simulink model "clawbot_planner"  (R2020b)
settings: Solver=VariableStepAuto  StartTime=0.0  StopTime=100  MaxStep=0.1  RelTol=1e-3
model workspace (MAT data in the model file):
  objPose = [-3 -4 0]
  pickup = 1
undefined symbols (not defined in the file): boxPose, goalPose, n_box, startPose, waypoints, X, Y, Z
libraries: sm_lib x10, robotics_pg_exp_pack x6, nesl_utility x5
settings Model: PacingRate=2  OrderedModelArguments=off  Creator=fciriell  LastModifiedBy=philip
settings ExplorerConfigSet: InternalSimMechanicsExplorerSettings="<ExplorerConfiguration><canonicalview>default</canonicalview><AnimationSetting><BasePlaybackSpeed>1.0</BasePlaybackSpeed><PlaybackSpeedFactor>1.0</PlaybackSpeedFactor></AnimationSetting><TilePanel><TileInfo><Tiles Columns=\"2\" Count=\"2\" Rows=\"1\"><Column Weight=\"0.4995\"/><Column Weight=\"0.5005\"/><Row Weight=\"1\"/><Tile Height=\"1\" Width=\"1\" X=\"0\" Y=\"0\"/><Tile Height=\"1\" Width=\"1\" X=\"1\" Y=\"0\"/></Tiles></TileInfo><SceneInfo><SceneViewer><BGColor><R>0.800000011920928955</R><G>1</G><B>1</B></BGColor><Camera><DoPerspective>off</DoPerspective><Position><X>-2157.55283921657792</X><Y>-624.799824111750013</Y><Z>101.181168331954723</Z></Position><Center><X>0.446420361421132839</X><Y>8.2063001014053043</Y><Z>-0.139153976130387491</Z></Center><Up><X>-0.0243727538639528785</X><Y>0.238484651328139785</Y><Z>0.970840378203329246</Z></Up><ViewLimDist>1</ViewLimDist><YLim>1.44671838529622754</YLim><XLim>1.08018402928996848</XLim></Camera></SceneViewer><SceneViewer><BGColor><R>0.800000011920928955</R><G>1</G><B>1</B></BGColor><Camera><DoPerspective>on</DoPerspective><Position><X>4.31003215901698322</X><Y>10.0399967053635688</Y><Z>0.101600000000000093</Z></Position><Center><X>3.31158832209072962</X><Y>9.99016648666538565</Y><Z>0.126637048717288314</Z></Center><Up><X>0.02500592574512428</X><Y>0.0012479928289858</Y><Z>0.999686523962150853</Z></Up><ViewLimDist>1</ViewLimDist><YLim>0.466307658154998583</YLim><XLim>0.348165952817071078</XLim></Camera></SceneViewer></SceneInfo></TilePanel><MechEditorPanel><Cameras><Camera><Id>Camera1</Id><Value><Name>pov</Name><NativeCamera><PositionTrackingFeature>ClawBot_Kinematic_Model_with_spherical_contact_gripper.Chassis.Vehicle_Base.Frame2</PositionTrackingFeature><CenterTrackingFeature>ClawBot_Kinematic_Model_with_spherical_contact_gripper.Claw_Arm.Claw_Base.Claw_Mount.Frame1</CenterTrackingFeature><UpVectorTrackingFeature>ClawBot_Kinematic_Model_with_spherical_contact_gripper.Claw_Arm.Claw_Base.Claw_Mount.Frame1</UpVectorTrackingFeature><CenterTrackingOrigin>off</CenterTrackingOrigin><CenterTrackingDirection>+Y</CenterTrackingDirection><UpVectorTrackingDirection>+X</UpVectorTrackingDirection></NativeCamera></Value></Camera><Camera><Id>Camera2</Id><Value><Name>topview</Name><NativeCamera><PositionKeyframeSet><Keyframe><Time>150</Time><Value><X>6.1546883145524589e-08</X><Y>-4.7109925072064129e-08</Y><Z>4.4114050188881766</Z></Value></Keyframe></PositionKeyframeSet><CenterKeyframeSet><Keyframe><Time>150</Time><Value><X>6.1546883145524589e-08</X><Y>-4.7109925072064129e-08</Y><Z>0.00050000002374872565</Z></Value></Keyframe></CenterKeyframeSet><UpVectorKeyframeSet><Keyframe><Time>150</Time><Value><X>0</X><Y>1</Y><Z>-0</Z></Value></Keyframe></UpVectorKeyframeSet></NativeCamera></Value></Camera></Cameras><GfxPanelCameraMap><MapElement CameraMLId=\"Camera1\" GfxPanelIndex=\"1\"/></GfxPanelCameraMap><VideoCreator><PlaybackSpeedRatio>1.0</PlaybackSpeedRatio><FrameRate>30</FrameRate><VideoFormat>Motion JPEG AVI</VideoFormat><FrameSize>auto</FrameSize></VideoCreator></MechEditorPanel></ExplorerConfiguration>"

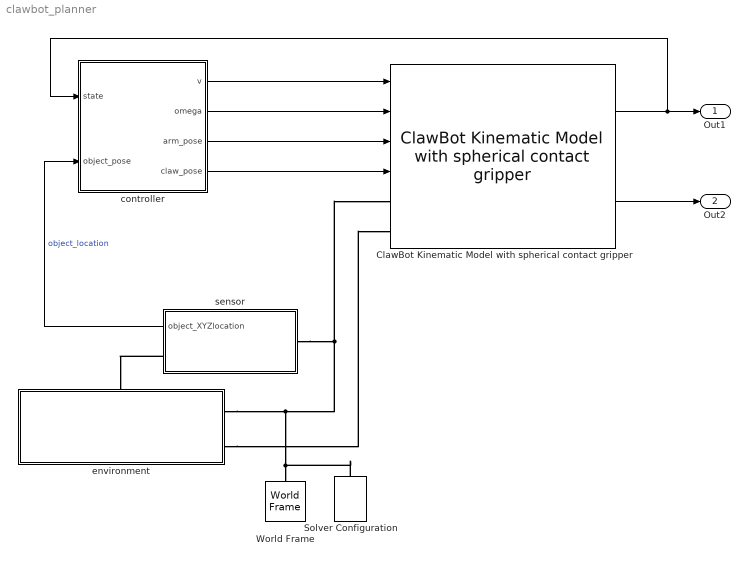
== system clawbot_planner ==
  ClawBot Kinematic Model with spherical contact gripper : robotics_pg_exp_pack/Robot Models/Clawbot/ClawBot Kinematic Model with spherical contact gripper  pose=startPose  k_contact=2*2.5*981  b_contact=sqrt(2*2.5*981)  x_contact=1e-2  u_statfric=10  u_dynfric=10  crit_vel_fric=1e-3  radius_contact_point=10  sensorTs=-1
      settings: SourceProductName=Robotics Playground Expansion Pack
  Solver Configuration : nesl_utility/Solver Configuration  PhysicalDomain=network_engine_domain  SubClassName=solver  LeftPortType=input  RightPortType=generic  Tones=[]  Harmonics=[]  SimulateNoise=off  Profile=off  UseLocalSampling=off  EnableSwitchedLinearOptims=on  FrequencyDomain=off  UseCCode=off  RelTol=0.001  AbsTol=1e-06  MinStep=1e-09  ToWorkspace=off  RevertToSquareIcSolve=off  NumHomotopyIterations=100  PhasorMode=off  PhasorModeNumHarmonics=1  DoDC=off  ResidualTolerance=1e-09  UseLocalSolver=off  LocalSolverChoice=NE_BACKWARD_EULER_ADVANCER  LocalSolverSampleTime=0.001  DoFixedCost=off  MaxNonlinIter=3  MaxModeIter=2  ComputeImpulses=off  ImpulseIterations=2  LinearAlgebra=auto  EquationFormulation=NE_TIME_EF  DelaysMemoryBudget=1024  AutomaticFiltering=on  FilteringTimeConstant=0.001  PartitionStorageMethod=AS_NEEDED  PartitionMemoryBudget=1024  PartitionMethod=ROBUST
  World Frame : sm_lib/Frames and Transforms/World Frame
  controller : Subsystem
  environment : Subsystem
      settings: PortSchema="{\"entries\":[{\"content\":{\"sides\":[{\"content\":{\"connectorIds\":[]},\"type\":\"ConnectorPlacement.EquallySpacedRectSide\",\"uuid\":\"883eba9b-41a6-4158-bc00-14a83777f32f\"},{\"content\":{\"connectorIds\":[\"RConn1\",\"RConn2\"],\"side\":\"RIGHT\"},\"type\":\"ConnectorPlacement.EquallySpacedRectSide\",\"uuid\":\"b95afd35-d391-4cad-9c3e-31548b5bac4e\"},{\"content\":{\"connectorIds\":[\"LConn1\"],\"side\":\"TOP\"},\"type\":\"ConnectorPlacement.EquallySpacedRectSide\",\"uuid\":\"0d35fa8f-0aa6-49ea-bb20-39be00b87579\"}]},\"type\":\"ConnectorPlacement.EquallySpacedConnector\",\"uuid\":\"10348ddd-2367-47d6-bad2-8db5a122cc9e\"}],\"packageUris\":[\"http://schema.mathworks.com/mf0/Connector/19700101\"],\"version\":\"1.0\"}"
  sensor : Subsystem
  Out1 : Outport
  Out2 : Outport  Port=2
  wires:
  sensor/1(object_XYZlocation) -> controller/2(object_pose)  "object_location"
  ClawBot Kinematic Model with spherical contact gripper/2 -> Out2/1
  ClawBot Kinematic Model with spherical contact gripper/1 -> controller/1(state), Out1/1
  controller/1(v) -> ClawBot Kinematic Model with spherical contact gripper/1
  controller/3(arm_pose) -> ClawBot Kinematic Model with spherical contact gripper/3
  controller/4(claw_pose) -> ClawBot Kinematic Model with spherical contact gripper/4
  controller/2(omega) -> ClawBot Kinematic Model with spherical contact gripper/2
  connections:
  environment/RConn1 -- Solver Configuration/RConn1 -- World Frame/RConn1 -- ClawBot Kinematic Model with spherical contact gripper/LConn1 -- sensor/LConn1
  environment/RConn2 -- ClawBot Kinematic Model with spherical contact gripper/LConn2
  sensor/RConn1 -- environment/LConn1

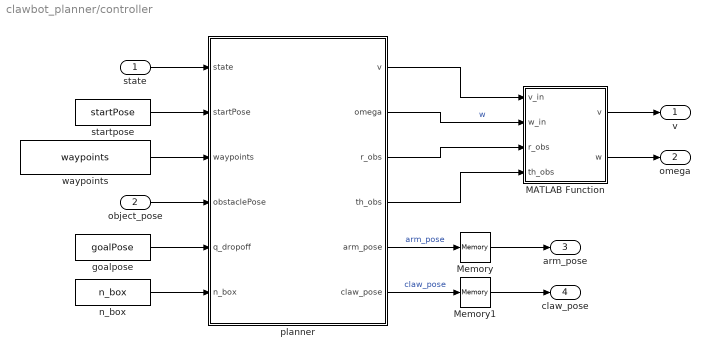
== system clawbot_planner/controller ==
  state : Inport
  object_pose : Inport  Port=2
  MATLAB Function : MATLAB Function  TreatAsAtomicUnit=on
  "Memory " : Memory
  Memory1 : Memory
  goalpose : Constant  Value=goalPose  SampleTime=0.01
  n_box : Constant  Value=n_box  SampleTime=0.01
  planner : Stateflow chart  TreatAsAtomicUnit=on
      settings: PortSchema="{\"entries\":[{\"content\":{\"sides\":[{\"content\":{\"connectorIds\":[\"In1\",\"In2\",\"In3\",\"In4\",\"In5\",\"In6\"]},\"type\":\"ConnectorPlacement.EquallySpacedRectSide\",\"uuid\":\"4907e7b4-59f6-4e30-9dc7-cd38531777e1\"},{\"content\":{\"connectorIds\":[\"Out1\",\"Out2\",\"Out6\",\"Out5\",\"Out3\",\"Out4\"],\"side\":\"RIGHT\"},\"type\":\"ConnectorPlacement.EquallySpacedRectSide\",\"uuid\":\"27f4ca00-c645-4624-ac98-a2a144dd84bb\"},{\"content\":{\"connectorIds\":[],\"side\":\"TOP\"},\"type\":\"ConnectorPlacement.EquallySpacedRectSide\",\"uuid\":\"2e3861bb-acf9-4584-a82a-efca55bff57a\"},{\"content\":{\"connectorIds\":[],\"side\":\"HIDDEN\"},\"type\":\"ConnectorPlacement.EquallySpacedRectSide\",\"uuid\":\"c95c31ea-85f8-4402-96cd-52bc89f7c1df\"}]},\"type\":\"ConnectorPlacement.EquallySpacedConnector\",\"uuid\":\"fce2e92a-f6ab-431e-a92c-b0146e5459eb\"}],\"packageUris\":[\"http://schema.mathworks.com/mf0/Connector/R2020b\"],\"version\":\"1.0\"}"
  startpose : Constant  Value=startPose  SampleTime=0.01
  waypoints : Constant  Value=waypoints  SampleTime=0.01
  v : Outport
  omega : Outport  Port=2
  arm_pose : Outport  Port=3
  claw_pose : Outport  Port=4
  wires:
  planner/4(claw_pose) -> Memory1/1  "claw_pose"
  planner/3(arm_pose) -> "Memory "/1  "arm_pose"
  Memory1/1 -> claw_pose/1
  "Memory "/1 -> arm_pose/1
  planner/1(v) -> MATLAB Function/1(v_in)
  goalpose/1 -> planner/5(q_dropoff)
  state/1 -> planner/1(state)
  startpose/1 -> planner/2(startPose)
  waypoints/1 -> planner/3(waypoints)
  object_pose/1 -> planner/4(obstaclePose)
  n_box/1 -> planner/6(n_box)
  MATLAB Function/2(w) -> omega/1
  planner/5(th_obs) -> MATLAB Function/4(th_obs)
  planner/6(r_obs) -> MATLAB Function/3(r_obs)
  planner/2(omega) -> MATLAB Function/2(w_in)  "w"
  MATLAB Function/1(v) -> v/1

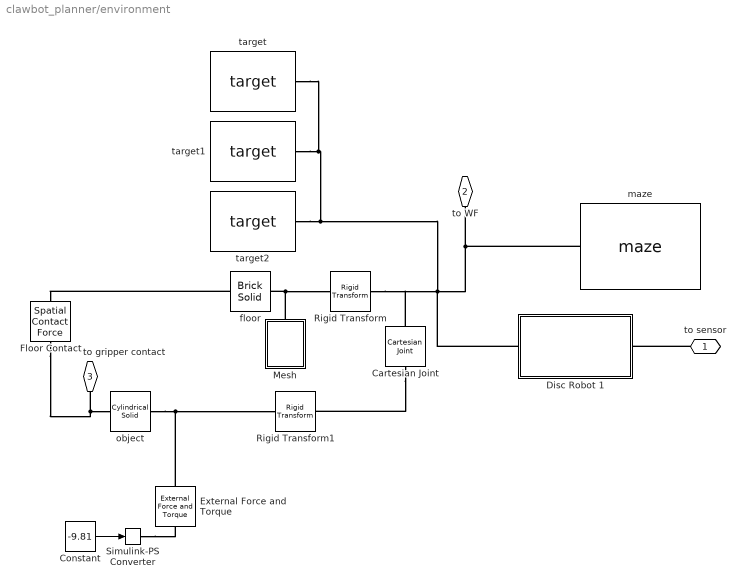
== system clawbot_planner/environment ==
  Cartesian Joint : sm_lib/Joints/Cartesian Joint  JointMode=Normal  SenseConstraintForce=off  SenseConstraintForceX=off  SenseConstraintForceY=off  SenseConstraintForceZ=off  SenseConstraintTorque=off  SenseConstraintTorqueX=off  SenseConstraintTorqueY=off  SenseConstraintTorqueZ=off  SenseTotalForce=off  SenseTotalForceX=off  SenseTotalForceY=off  SenseTotalForceZ=off  SenseTotalTorque=off  SenseTotalTorqueX=off  SenseTotalTorqueY=off  SenseTotalTorqueZ=off  CompositeWrenchDir=FollowerOnBase  CompositeWrenchFrame=BaseFrame  PxEquilibriumPosition=0  PxEquilibriumPositionUnits=m  PxSpringStiffness=1e-1  PxSpringStiffnessUnits=N/m  PxDampingCoefficient=1e-2  PxDampingCoefficientUnits=N/(m/s)  PxTorqueActuationMode=NoTorque  PxMotionActuationMode=ComputedMotion  PxSensePosition=off  PxSenseVelocity=off  PxSenseAcceleration=off  PxSenseTorqueForce=off  PxSenseLowerLimitTorqueForce=off  PxSenseUpperLimitTorqueForce=off  PxLowerLimitSpecify=off  PxLowerLimitBound=-1  PxLowerLimitBoundUnits=m  PxLowerLimitStiffness=1e6  PxLowerLimitStiffnessUnits=N/m  PxLowerLimitDamping=1e3  PxLowerLimitDampingUnits=N/(m/s)  PxLowerLimitTransitionRegionWidth=1e-4  PxLowerLimitTransitionRegionWidthUnits=m  PxUpperLimitSpecify=off  PxUpperLimitBound=1  PxUpperLimitBoundUnits=m  PxUpperLimitStiffness=1e6  PxUpperLimitStiffnessUnits=N/m  PxUpperLimitDamping=1e3  PxUpperLimitDampingUnits=N/(m/s)  PxUpperLimitTransitionRegionWidth=1e-4  PxUpperLimitTransitionRegionWidthUnits=m  PxPositionTargetSpecify=off  PxPositionTargetPriority=High  PxPositionTargetValue=0  PxPositionTargetValueUnits=m  PxVelocityTargetSpecify=off  PxVelocityTargetPriority=High  PxVelocityTargetValue=0  PxVelocityTargetValueUnits=m/s  PyEquilibriumPosition=0  PyEquilibriumPositionUnits=m  PySpringStiffness=1e-1  PySpringStiffnessUnits=N/m  PyDampingCoefficient=1e-2  PyDampingCoefficientUnits=N/(m/s)  PyTorqueActuationMode=NoTorque  PyMotionActuationMode=ComputedMotion  PySensePosition=off  PySenseVelocity=off  PySenseAcceleration=off  PySenseTorqueForce=off  PySenseLowerLimitTorqueForce=off  PySenseUpperLimitTorqueForce=off  PyLowerLimitSpecify=off  PyLowerLimitBound=-1  PyLowerLimitBoundUnits=m  PyLowerLimitStiffness=1e6  PyLowerLimitStiffnessUnits=N/m  PyLowerLimitDamping=1e3  PyLowerLimitDampingUnits=N/(m/s)  PyLowerLimitTransitionRegionWidth=1e-4  PyLowerLimitTransitionRegionWidthUnits=m  PyUpperLimitSpecify=off  PyUpperLimitBound=1  PyUpperLimitBoundUnits=m  PyUpperLimitStiffness=1e6  PyUpperLimitStiffnessUnits=N/m  PyUpperLimitDamping=1e3  PyUpperLimitDampingUnits=N/(m/s)  PyUpperLimitTransitionRegionWidth=1e-4  PyUpperLimitTransitionRegionWidthUnits=m  PyPositionTargetSpecify=off  PyPositionTargetPriority=High  PyPositionTargetValue=0  PyPositionTargetValueUnits=m  PyVelocityTargetSpecify=off  PyVelocityTargetPriority=High  PyVelocityTargetValue=0  PyVelocityTargetValueUnits=m/s  PzEquilibriumPosition=0  PzEquilibriumPositionUnits=m  PzSpringStiffness=1e-1  PzSpringStiffnessUnits=N/m  PzDampingCoefficient=1e-2  PzDampingCoefficientUnits=N/(m/s)  PzTorqueActuationMode=NoTorque  PzMotionActuationMode=ComputedMotion  PzSensePosition=off  PzSenseVelocity=off  PzSenseAcceleration=off  PzSenseTorqueForce=off  PzSenseLowerLimitTorqueForce=off  PzSenseUpperLimitTorqueForce=off  PzLowerLimitSpecify=off  PzLowerLimitBound=-1  PzLowerLimitBoundUnits=m  PzLowerLimitStiffness=1e6  PzLowerLimitStiffnessUnits=N/m  PzLowerLimitDamping=1e3  PzLowerLimitDampingUnits=N/(m/s)  PzLowerLimitTransitionRegionWidth=1e-4  PzLowerLimitTransitionRegionWidthUnits=m  PzUpperLimitSpecify=off  PzUpperLimitBound=1  PzUpperLimitBoundUnits=m  PzUpperLimitStiffness=1e6  PzUpperLimitStiffnessUnits=N/m  PzUpperLimitDamping=1e3  PzUpperLimitDampingUnits=N/(m/s)  PzUpperLimitTransitionRegionWidth=1e-4  PzUpperLimitTransitionRegionWidthUnits=m  PzPositionTargetSpecify=off  PzPositionTargetPriority=High  PzPositionTargetValue=0  PzPositionTargetValueUnits=m  PzVelocityTargetSpecify=off  PzVelocityTargetPriority=High  PzVelocityTargetValue=0  PzVelocityTargetValueUnits=m/s
  Constant : Constant  Value=-9.81
  Disc Robot 1 : Subsystem
  External Force and Torque : sm_lib/Forces and Torques/External Force and Torque  ForceResolutionFrame=AttachedFrame  EnableForceX=off  EnableForceY=off  EnableForceZ=on  EnableForce=off  TorqueResolutionFrame=AttachedFrame  EnableTorqueX=off  EnableTorqueY=off  EnableTorqueZ=off  EnableTorque=off
  "Floor Contact  " : sm_lib/Forces and Torques/Spatial Contact Force  CoefficientOfDynamicFriction=0.3  CoefficientOfStaticFriction=0.5  NormalDamping=1e3  NormalDampingUnits=N/(m/s)  NormalStiffness=1e6  NormalStiffnessUnits=N/m  FrictionalCriticalVelocity=1e-3  FrictionalCriticalVelocityUnits=m/s  ZeroCrossDetectContactStartAndEnd=off  SenseFrictionalForceMagnitude=off  SenseNormalForceMagnitude=off  SenseSeparationDistance=off  NormalTransitionRegionWidth=1e-4  NormalTransitionRegionWidthUnits=m  FrictionType=SmoothStickSlip
  "Mesh " : Subsystem  mask(Rectangular Mesh){mesh_lenx=20, mesh_leny=20, mesh_hx=0.1, mesh_hy=0.1, mesh_numhx=29, mesh_numhy=29, mesh_thickness=0.01, mesh_rho=7000, mesh_color=[0 0.4 0.6], mesh_opc=0.5}
      mask prompts: mesh_thickness "Thickness (m)"; mesh_rho "Density (kg/m^3)"; mesh_color "Color [RGB]"; mesh_opc "Opacity (0-1)"
      mask help: Rectangular mesh. Define outer dimensions, dimensions of holes, and thickness. R port is at the CG. Thickness defines the distance of the F frame from the B frame along the z-axis.
      mask init:
      | mesh_xsec = Extr_Data_Mesh(mesh_lenx, mesh_leny, mesh_numhx, mesh_numhy, mesh_hx, mesh_hy);
      mask DialogControl Control12 Prompt: Plot Profile
      mask DialogControl Control12 Callback:
      | v = get_param(gcb,'MaskWSVariables');
      | getMaskValue = containers.Map({v.Name}',{v.Value}');
      | evalin('base',...
      |     sprintf('Extr_Data_Mesh(%s,%s,%s,%s,%s,%s,''%s'');',...
      |     num2str(getMaskValue('mesh_lenx')),...
      |     num2str(getMaskValue('mesh_leny')),...
      |     num2str(getMaskValue('mesh_numhx')),...
      |     num2str(getMaskValue('mesh_numhy')),...
      |     num2str(getMaskValue('mesh_hx')),...
      |     num2str(getMaskValue('mesh_hy')),'plot'));
      mask DialogControl Control7 Prompt: X
      mask DialogControl Control8 Prompt: Y
      mask DialogControl Control9 Prompt: Mesh Length (m)
      mask DialogControl Control11 Prompt: Hole Length (m)
      mask DialogControl Control10 Prompt: Number of Holes
  Rigid Transform : sm_lib/Frames and Transforms/Rigid Transform  TranslationMethod=Cartesian  TranslationStandardOffset=0  TranslationLengthUnit=m  TranslationStandardAxis=+Z  TranslationCartesianOffset=[-10 -10 0]  TranslationROffset=0  TranslationROffsetUnits=m  TranslationZOffset=0  TranslationZOffsetUnits=m  TranslationThetaOffset=0  TranslationThetaOffsetUnits=deg  RotationMethod=None  RotationAngleUnits=deg  RotationStandardAxis=+Z  RotationAngle=0.0  RotationArbitraryAxis=[0 0 1]  FollAlignAxisA=+X  BaseAlignAxisA=+Y  FollAlignAxisB=+Y  BaseAlignAxisB=+Z  RotationSequenceAxes=FollowerAxes  RotationSequence=XYX  RotationSequenceAngles=[0 0 0]  RotationSequenceAnglesUnits=deg  RotationMatrix=[1 0 0; 0 1 0; 0 0 1]
      settings: AttributesFormatString=XYZ = %<TranslationCartesianOffset>
  Rigid Transform1 : sm_lib/Frames and Transforms/Rigid Transform  TranslationMethod=Cartesian  TranslationStandardOffset=0  TranslationLengthUnit=m  TranslationStandardAxis=+Z  TranslationCartesianOffset=[-boxPose(1) -boxPose(2) 0]  TranslationROffset=0  TranslationROffsetUnits=m  TranslationZOffset=0  TranslationZOffsetUnits=m  TranslationThetaOffset=0  TranslationThetaOffsetUnits=deg  RotationMethod=None  RotationAngleUnits=deg  RotationStandardAxis=+Z  RotationAngle=0.0  RotationArbitraryAxis=[0 0 1]  FollAlignAxisA=+X  BaseAlignAxisA=+Y  FollAlignAxisB=+Y  BaseAlignAxisB=+Z  RotationSequenceAxes=FollowerAxes  RotationSequence=XYX  RotationSequenceAngles=[0 0 0]  RotationSequenceAnglesUnits=deg  RotationMatrix=[1 0 0; 0 1 0; 0 0 1]
      settings: AttributesFormatString=XYZ = %<TranslationCartesianOffset>
  Simulink-PS Converter : nesl_utility/Simulink-PS Converter  PhysicalDomain=network_engine_domain  SubClassName=ps_input  LeftPortType=input  RightPortType=output  PseudoPeriodic=off  Frequencies=[]  NoiseDistribution=none  NoiseParameters=[]  Unit=1  AffineConversion=off  FilteringAndDerivatives=provide  SimscapeFilterOrder=1  InputFilterTimeConstant=0.001  UdotUserProvided=0
  floor : sm_lib/Body Elements/Brick Solid  GraphicAmbientColor=[0.15 0.15 0.15 1.0]  BasedOnType=Density  BrickDimensions=[20 20 0.01]  BrickDimensionUnits=m  CenterOfMass=[0 0 0]  CenterOfMassUnits=m  GraphicDiffuseColor=[1.0 1.0 1.0]  Density=1000  DensityUnits=kg/m^3  DoExposeReferenceFrame=off  GraphicEmissiveColor=[0.0 0.0 0.0 1.0]  ExportEntireGeometry=on  SerializedFrames=<Frames><Frame><Id>Frame1</Id><Value><Name>TF</Name><Origin><Source>ReferenceFrame</Source><FeatureName></FeatureName></Origin><PrimaryAxis><DefinedDirection>+Z</DefinedDirection><Source>ReferenceFrame</Source><SourceDirection>+Z</SourceDirection><FeatureName></FeatureName></PrimaryAxis><SecondaryAxis><DefinedDirection>+X</DefinedDirection><Source>ReferenceFrame</Source><SourceDirection>+X</SourceDirection><FeatureName></FeatureName></SecondaryAxis></Value></Frame></Frames>  MarkerShape=Sphere  MarkerSize=10  GraphicType=FromGeometry  InertiaType=CalculateFromGeometry  Mass=1  MassUnits=kg  MomentsOfInertia=[1 1 1]  MomentsOfInertiaUnits=kg*m^2  GraphicOpacity=1.0  ProductsOfInertia=[0 0 0]  ProductsOfInertiaUnits=kg*m^2  GraphicShininess=75  GraphicSpecularColor=[0.5 0.5 0.5 1.0]  GraphicVisPropType=SimpleVisualProperties
  maze : robotics_pg_exp_pack/Environments & Sensors/Simscape Multibody Environments/maze  map=maze  wall_height=2  resolution=resolution  branching=branching
      link override File Solid: SerializedFrames=<Frames><Frame><Id>Frame1</Id><Value><Name>F1</Name><Origin><Source>ReferenceFrame</Source><FeatureName></FeatureName></Origin><PrimaryAxis><DefinedDirection>+Z</DefinedDirection><Source>ReferenceFrame</Source><SourceDirection>+Z</SourceDirection><FeatureName></FeatureName></PrimaryAxis><SecondaryAxis><DefinedDirection>+X</DefinedDirection><Source>ReferenceFrame</Source><SourceDirection>+X</SourceDirection><FeatureName></FeatureName></SecondaryAxis></Value></Frame></Frames>
      settings: SourceProductName=Robotics Playground Expansion Pack
  object : sm_lib/Body Elements/Cylindrical Solid  GraphicAmbientColor=[0.15 0.15 0.15 1.0]  BasedOnType=Density  CenterOfMass=[0 0 0]  CenterOfMassUnits=m  GraphicDiffuseColor=[0.0 1.0 1.0]  CylinderLength=300  CylinderLengthUnits=mm  CylinderRadius=20  CylinderRadiusUnits=mm  Density=1000  DensityUnits=kg/m^3  DoExposeReferenceFrame=off  GraphicEmissiveColor=[0.0 0.0 0.0 1.0]  ExportEntireGeometry=on  SerializedFrames=<Frames><Frame><Id>Frame1</Id><Value><Name>BF</Name><Origin><Source>GeometricFeature</Source><FeatureName>bottom surface</FeatureName></Origin><PrimaryAxis><DefinedDirection>+Z</DefinedDirection><Source>ReferenceFrame</Source><SourceDirection>+Z</SourceDirection><FeatureName></FeatureName></PrimaryAxis><SecondaryAxis><DefinedDirection>+X</DefinedDirection><Source>ReferenceFrame</Source><SourceDirection>+X</SourceDirection><FeatureName></FeatureName></SecondaryAxis></Value></Frame></Frames>  MarkerShape=Sphere  MarkerSize=10  GraphicType=FromGeometry  InertiaType=PointMass  Mass=1  MassUnits=kg  MomentsOfInertia=[1 1 1]  MomentsOfInertiaUnits=kg*m^2  GraphicOpacity=0.8  ProductsOfInertia=[0 0 0]  ProductsOfInertiaUnits=kg*m^2  GraphicShininess=75  GraphicSpecularColor=[0.5 0.5 0.5 1.0]  GraphicVisPropType=SimpleVisualProperties
      settings: AttributesFormatString=mass = %<Mass> kg
  target : robotics_pg_exp_pack/Environments & Sensors/Simscape Multibody Environments/target  pose=boxPose  color=[0.5 0.2 0.2]  radiusTarget=0.5
      link override Rigid Transform2: TranslationCartesianOffset=[-boxPose(1) -boxPose(2) -0.01]
      link override Rigid Transform4: RotationAngle=startPose(3)
      settings: SourceProductName=Robotics Playground Expansion Pack
  target1 : robotics_pg_exp_pack/Environments & Sensors/Simscape Multibody Environments/target  pose=[startPose]  color=[0.2 0.5 0.2]  radiusTarget=0.5
      link override Rigid Transform2: TranslationCartesianOffset=[-startPose(1) -startPose(2) -0.01]
      link override Rigid Transform4: RotationAngle=startPose(3)
      settings: SourceProductName=Robotics Playground Expansion Pack
  target2 : robotics_pg_exp_pack/Environments & Sensors/Simscape Multibody Environments/target  pose=[goalPose]  color=[0.2 0.2 0.5]  radiusTarget=0.5
      link override Rigid Transform2: TranslationCartesianOffset=[-goalPose(1) -goalPose(2) -0.01]
      link override Rigid Transform4: RotationAngle=goalPose(3)
      settings: SourceProductName=Robotics Playground Expansion Pack
  to sensor : PMIOPort  Side=Left
  "to WF " : PMIOPort  Port=2  Side=Right
  to gripper contact : PMIOPort  Port=3  Side=Right
  wires:
  Constant/1 -> Simulink-PS Converter/1
  connections:
  Cartesian Joint/RConn1 -- Rigid Transform1/RConn1
  "Floor Contact  "/LConn1 -- to gripper contact/RConn1 -- object/RConn1
  object/LConn1 -- External Force and Torque/RConn1 -- Rigid Transform1/LConn1
  floor/RConn1 -- "Floor Contact  "/RConn1
  Simulink-PS Converter/RConn1 -- External Force and Torque/LConn1
  "Mesh "/LConn1 -- Rigid Transform/LConn1 -- floor/LConn1
  target/LConn1 -- Disc Robot 1/LConn1 -- Rigid Transform/RConn1 -- Cartesian Joint/LConn1 -- maze/RConn1 -- "to WF "/RConn1 -- target2/LConn1 -- target1/LConn1
  to sensor/RConn1 -- Disc Robot 1/RConn1

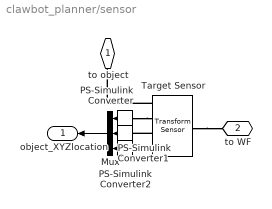
== system clawbot_planner/sensor ==
  Mux : Mux  Inputs=3
  PS-Simulink Converter : nesl_utility/PS-Simulink Converter  PhysicalDomain=network_engine_domain  SubClassName=ps_output  LeftPortType=input  RightPortType=output  PseudoPeriodic=off  Frequencies=[]  Unit=inherit  AffineConversion=off
  PS-Simulink Converter1 : nesl_utility/PS-Simulink Converter  PhysicalDomain=network_engine_domain  SubClassName=ps_output  LeftPortType=input  RightPortType=output  PseudoPeriodic=off  Frequencies=[]  Unit=inherit  AffineConversion=off
  PS-Simulink Converter2 : nesl_utility/PS-Simulink Converter  PhysicalDomain=network_engine_domain  SubClassName=ps_output  LeftPortType=input  RightPortType=output  PseudoPeriodic=off  Frequencies=[]  Unit=inherit  AffineConversion=off
  "Target Sensor " : sm_lib/Frames and Transforms/Transform Sensor  MeasurementFrame=World  SenseAngle=off  SenseAxis=off  SenseAngle1=off  SenseAngle2=off  SenseAngle3=off  SenseQ=off  SenseR=off  SenseOmegaX=off  SenseOmegaY=off  SenseOmegaZ=off  SenseOmega1=off  SenseOmega2=off  SenseOmega3=off  SenseQDot=off  SenseRDot=off  SenseAlphaX=off  SenseAlphaY=off  SenseAlphaZ=off  SenseAlpha1=off  SenseAlpha2=off  SenseAlpha3=off  SenseQDDot=off  SenseRDDot=off  SenseX=on  SenseY=on  SenseZ=on  SenseRad=off  SenseAzim=off  SenseDist=off  SenseInc=off  SenseXDot=off  SenseYDot=off  SenseZDot=off  SenseRadDot=off  SenseAzimDot=off  SenseDistDot=off  SenseIncDot=off  SenseXDDot=off  SenseYDDot=off  SenseZDDot=off  SenseRadDDot=off  SenseAzimDDot=off  SenseDistDDot=off  SenseIncDDot=off
  to object : PMIOPort  Side=Right
  to WF : PMIOPort  Port=2  Side=Left
  object_XYZlocation : Outport
  wires:
  Mux/1 -> object_XYZlocation/1
  PS-Simulink Converter2/1 -> Mux/3
  PS-Simulink Converter/1 -> Mux/1
  PS-Simulink Converter1/1 -> Mux/2
  connections:
  "Target Sensor "/RConn1 -- to object/RConn1
  "Target Sensor "/LConn1 -- to WF/RConn1
  "Target Sensor "/RConn4 -- PS-Simulink Converter2/LConn1
  "Target Sensor "/RConn3 -- PS-Simulink Converter1/LConn1
  PS-Simulink Converter/LConn1 -- "Target Sensor "/RConn2

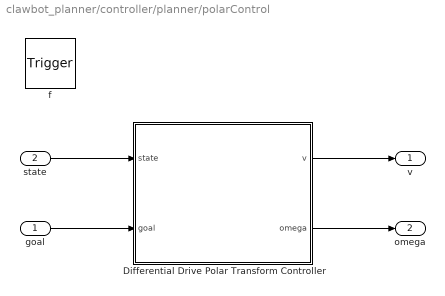
== system clawbot_planner/controller/planner/polarControl ==
  goal : Inport  OutDataTypeStr=double  PortDimensions=3
  state : Inport  Port=2  OutDataTypeStr=double  PortDimensions=3
  f : TriggerPort  TriggerType=function-call  VariantControl=(inherit)
      settings: CopyFcn=Stateflow.SLINSF.SimulinkMan.removeBlockPreDeleteFcn  PreDeleteFcn=Stateflow.SLINSF.SimulinkMan.unsafePredeleteFcn
  Differential Drive Polar Transform Controller : Subsystem  AncestorBlock=robotics_pg_exp_pack/Controllers/Differential Drive Polar Transform Controller  mask(controller){krho=1, kalpha=3, kbeta=-0.1}
      mask help:
      | A proportional controller that uses a polar transformation to control a differential drive robot towards a target pose.
      |
      | Inputs:
      | - q_goal =  [x_goal y_goal theta_goal]
      | - state    =  [x y theta]
      |
      | Outputs:
      | - v, linear velocity
      | - omega, angular velocity
      |
      | The behaviour of the controller can be modified by the gain parameters, krho, kalpha, kbeta.
      |
      | For robust position control,
      |
      | krho > 0
      | kbeta < 0
      | kalpha + 5/3 * kbeta - 2/pi * krho > 0
      mask Display: image('$imagefile', [0.2 0.1 0.6 0.8]); % Use "Edit Image" on toolstrip to change.
  v : Outport
  omega : Outport  Port=2
  wires:
  Differential Drive Polar Transform Controller/1(v) -> v/1
  Differential Drive Polar Transform Controller/2(omega) -> omega/1
  state/1 -> Differential Drive Polar Transform Controller/1(state)
  goal/1 -> Differential Drive Polar Transform Controller/2(goal)

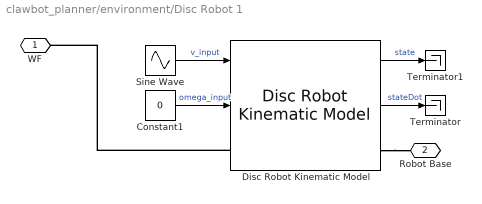
== system clawbot_planner/environment/Disc Robot 1 ==
  Constant1 : Constant  Value=0
  Disc Robot Kinematic Model : robotics_pg_exp_pack/Robot Models/MATLAB Disc Robot/Disc Robot Kinematic Model  wheelRadius=0.1  wheelBase=0.5  wheelThickness=0.025  chassisThickness=0.05  startPose=disc1StartPose  choice=off  sensorTs=0.05  wheelColor=[0.25 0.25 0.25]  chassisColor=[0.5 0.25 0.25]
      settings: SourceProductName=Robotics Playground Expansion Pack
  Sine Wave : Sin  Amplitude=3.8  Frequency=pi/7  SampleTime=0
  Terminator : Terminator
  Terminator1 : Terminator
  WF : PMIOPort  Side=Left
  Robot Base : PMIOPort  Port=2  Side=Right
  wires:
  Constant1/1 -> Disc Robot Kinematic Model/2  "omega_input"
  Sine Wave/1 -> Disc Robot Kinematic Model/1  "v_input"
  Disc Robot Kinematic Model/1 -> Terminator1/1  "state"
  Disc Robot Kinematic Model/2 -> Terminator/1  "stateDot"
  connections:
  Disc Robot Kinematic Model/LConn1 -- WF/RConn1
  Disc Robot Kinematic Model/RConn1 -- Robot Base/RConn1

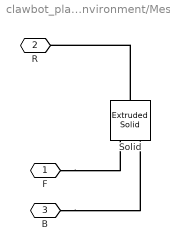
== system clawbot_planner/environment/Mesh  ==
  Solid : sm_lib/Body Elements/Extruded Solid  GraphicAmbientColor=[0.15 0.15 0.15 1.0]  BasedOnType=Density  CenterOfMass=[0 0 0]  CenterOfMassUnits=m  GraphicDiffuseColor=mesh_color  ExportConvexHullGeometry=off  ExtrusionCrossSection=mesh_xsec  ExtrusionCrossSectionUnits=m  Density=mesh_rho  DensityUnits=kg/(m^3)  DoExposeReferenceFrame=on  GraphicEmissiveColor=[0.0 0.0 0.0 1.0]  ExportEntireGeometry=off  ExtrusionLength=mesh_thickness  ExtrusionLengthUnits=m  ExtrusionType=General  SerializedFrames=<Frames><Frame><Id>Frame1</Id><Value><Name>F</Name><Origin><Source>GeometricFeature</Source><FeatureName>top surface</FeatureName></Origin><PrimaryAxis><DefinedDirection>+Z</DefinedDirection><Source>ReferenceFrame</Source><SourceDirection>+Z</SourceDirection><FeatureName></FeatureName></PrimaryAxis><SecondaryAxis><DefinedDirection>+X</DefinedDirection><Source>ReferenceFrame</Source><SourceDirection>+X</SourceDirection><FeatureName></FeatureName></SecondaryAxis></Value></Frame><Frame><Id>Frame2</Id><Value><Name>B</Name><Origin><Source>GeometricFeature</Source><FeatureName>bottom surface</FeatureName></Origin><PrimaryAxis><DefinedDirection>+Z</DefinedDirection><Source>ReferenceFrame</Source><SourceDirection>+Z</SourceDirection><FeatureName></FeatureName></PrimaryAxis><SecondaryAxis><DefinedDirection>+X</DefinedDirection><Source>ReferenceFrame</Source><SourceDirection>+X</SourceDirection><FeatureName></FeatureName></SecondaryAxis></Value></Frame></Frames>  MarkerShape=Sphere  MarkerSize=10  GraphicType=FromGeometry  InertiaType=CalculateFromGeometry  Mass=1  MassUnits=kg  MomentsOfInertia=[1 1 1]  MomentsOfInertiaUnits=kg*m^2  PolygonNumSides=3  GraphicOpacity=mesh_opc  PolygonOuterRadius=1  PolygonOuterRadiusUnits=m  ProductsOfInertia=[0 0 0]  ProductsOfInertiaUnits=kg*m^2  GraphicShininess=75  GraphicSpecularColor=[0.5 0.5 0.5 1.0]  GraphicVisPropType=SimpleVisualProperties
  F : PMIOPort  Side=Right
  R : PMIOPort  Port=2  Side=Left
  B : PMIOPort  Port=3  Side=Right
  connections:
  B/RConn1 -- Solid/LConn2
  F/RConn1 -- Solid/LConn1
  Solid/RConn1 -- R/RConn1

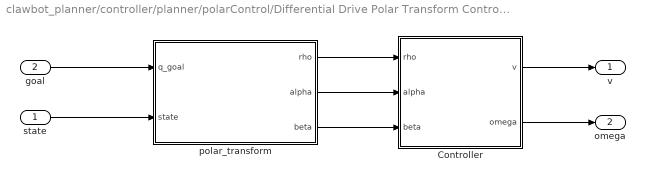
== system clawbot_planner/controller/planner/polarControl/Differential Drive Polar Transform Controller ==
  state : Inport
  goal : Inport  Port=2
  Controller : Subsystem
  polar_transform : Subsystem
  v : Outport
  omega : Outport  Port=2
  wires:
  polar_transform/3(beta) -> Controller/3(beta)
  polar_transform/2(alpha) -> Controller/2(alpha)
  polar_transform/1(rho) -> Controller/1(rho)
  state/1 -> polar_transform/2(state)
  goal/1 -> polar_transform/1(q_goal)
  Controller/1(v) -> v/1
  Controller/2(omega) -> omega/1

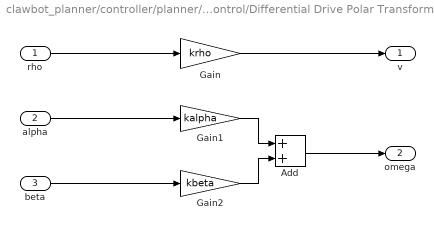
== system clawbot_planner/controller/planner/polarControl/Differential Drive Polar Transform Controller/Controller ==
  rho : Inport
  alpha : Inport  Port=2
  beta : Inport  Port=3
  Add : Sum
  Gain : Gain  Gain=krho
  Gain1 : Gain  Gain=kalpha
  Gain2 : Gain  Gain=kbeta
  v : Outport
  omega : Outport  Port=2
  wires:
  beta/1 -> Gain2/1
  Add/1 -> omega/1
  Gain1/1 -> Add/1
  rho/1 -> Gain/1
  Gain/1 -> v/1
  alpha/1 -> Gain1/1
  Gain2/1 -> Add/2

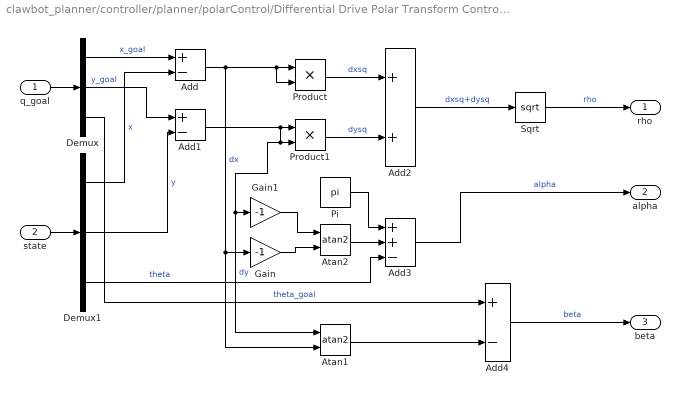
== system clawbot_planner/controller/planner/polarControl/Differential Drive Polar Transform Controller/polar_transform ==
  q_goal : Inport
  state : Inport  Port=2
  Add : Sum  Inputs=+-
  Add1 : Sum  Inputs=+-
  Add2 : Sum
  Add3 : Sum  Inputs=++-
  Add4 : Sum  Inputs=+-
  Atan1 : Trigonometry  Operator=atan2
  Atan2 : Trigonometry  Operator=atan2
  Demux : Demux  Outputs=3
  Demux1 : Demux  Outputs=3
  Gain : Gain  Gain=-1
  Gain1 : Gain  Gain=-1
  Pi : Constant  Value=pi  OutDataTypeStr=Inherit: Inherit via back propagation
  Product : Product
  Product1 : Product
  Sqrt : Sqrt  SaturateOnIntegerOverflow=on
  rho : Outport
  alpha : Outport  Port=2
  beta : Outport  Port=3
  wires:
  Add4/1 -> beta/1  "beta"
  Sqrt/1 -> rho/1  "rho"
  state/1 -> Demux1/1
  Demux1/2 -> Add1/2  "y"
  q_goal/1 -> Demux/1
  Atan2/1 -> Add3/2
  Demux/3 -> Add4/1  "theta_goal"
  Demux1/1 -> Add/2  "x"
  Add2/1 -> Sqrt/1  "dxsq+dysq"
  Product1/1 -> Add2/2  "dysq"
  Demux/1 -> Add/1  "x_goal"
  Add3/1 -> alpha/1  "alpha"
  Product/1 -> Add2/1  "dxsq"
  Demux/2 -> Add1/1  "y_goal"
  Add1/1 -> Atan1/1, Gain1/1, Product1/2, Product1/1  "dy"
  Demux1/3 -> Add3/3  "theta"
  Add/1 -> Product/1, Product/2, Atan1/2, Gain/1  "dx"
  Pi/1 -> Add3/1
  Gain/1 -> Atan2/2
  Gain1/1 -> Atan2/1
  Atan1/1 -> Add4/2

== matlab function clawbot_planner/controller/MATLAB Function ==
  data: v_in input; w_in input; r_obs input; v output; th_obs input; w output
function [v,w] = fcn(v_in, w_in, r_obs, th_obs)

if r_obs < 3 && th_obs < 0.5
    w = w_in - 5*sign(th_obs);
    v = v_in/2;
else
    v = v_in;
    w = w_in;
end

== stateflow chart clawbot_planner/controller/planner ==
  state Dropoff_lower_arm
    entry:
    arm_pose = -19
    v = 0
    omega = 0
  state Dropoff_open_claw
    entry:
    claw_pose = -20
  state Start
    entry:
    n=2;
    n_waypoints=size(waypoints,1);
    arm_pose = -30;
    claw_pose = -20;
    p = 1
  state ToGoal
    entry:
    error = inf;
    goal = waypoints(n,:)';
    claw_state = clawTransform(goal, state);
    %arm_pose = -30;
    %claw_pose = -20;
    %
    during:
    claw_state = clawTransform(goal, state);
    [v omega] = polarControl(goal, claw_state);
    dx = goal(1)-claw_state(1);
    dy = goal(2)-claw_state(2);
    dth = rem(goal(3)-claw_state(3),pi);
    error = sqrt(dx^2+dy^2+dth^2);
  state ToWaypoint
    entry:
    error = inf;
    goal = waypoints(n,:)';
    claw_state = clawTransform(goal, state);
    %arm_pose = -30;
    %claw_pose = -20;
    %
    during:
    claw_state = clawTransform(goal, state);
    [v omega] = polarControl(goal, claw_state);
    dx = goal(1)-claw_state(1);
    dy = goal(2)-claw_state(2);
    r_obs = norm(obstaclePose(1:2)-state(1:2));
    th_obs = atan2(obstaclePose(2)-state(2),obstaclePose(1)-state(1));
    error = sqrt(dx^2+dy^2);
  state NextWaypoint
    entry:
    n=n+1;
  state Todest
    entry:
    n_waypoints=size(waypoints,1);
    p = 0
  state Pickup
    entry:
    arm_pose = 15
    during:
    v = 0
    omega = 0
  state Close_gripper
    during:
    %claw_pose = claw_pose + 2
    claw_pose = 11
  state Raise_arm
    during:
    arm_pose = -30
  state [v,omega] = polarControl(goal, state) [function]
  Dropoff_lower_arm -> Dropoff_open_claw : [after(3,sec)]
  (default) -> Start
  ToGoal -> Dropoff_lower_arm [order 2] : [error<0.5&&p==0]
  Start -> ToWaypoint
  ToWaypoint -> NextWaypoint : [error<1]
  NextWaypoint -> ToGoal [order 1] : [n==n_waypoints]
  Todest -> ToWaypoint
  NextWaypoint -> ToWaypoint [order 4] : [n>n_box]{n_box<n<n_waypoints}
  NextWaypoint -> ToGoal [order 3] : [n==n_box]
  NextWaypoint -> ToWaypoint [order 2] : [n<n_box]{n<n_box}
  ToGoal -> Pickup [order 1] : [error<0.05&&p==1]
  Raise_arm -> Todest : [after(3,sec)]
  Close_gripper -> Raise_arm : [after(3,sec)]
  Pickup -> Close_gripper : [after(5,sec)]
  data: goal function_input double size=3; state function_input double size=3; v function_output; omega function_output; q function_input double size=3; s function_input double size=3; cs function_output double size=3; state input; startPose input; waypoints input; obstaclePose input; dx local; dth local; dy local; error local; n local; n_waypoints local; q_dropoff input; v output; omega output; claw_state local; goal local; arm_pose output; claw_pose output; n_box input; p local; th_obs output; r_obs output double
  function cs = clawTransform(q, s):
    | function cs = clawTransform(q, s)
    |  
    | cs = [s(1) + 0.3126*cos(0.1283 + q(3)); s(2) + 0.3126*sin(0.1283 + q(3)); s(3) ];
